simulink model "gm_sampleModel1973_sub_sub_sub"  (R2023a)
settings: Solver=VariableStepAuto  StartTime=0.0  StopTime=10.0  RelTol=1e-3
libraries: simulink x5, hdlsllib x4
settings Model: Creator=user1  LastModifiedBy=user1
settings OptimizationCC: BlockReduction=off  ConditionallyExecuteInputs=off
settings DebuggingCC: InheritedTsInSrcMsg=none

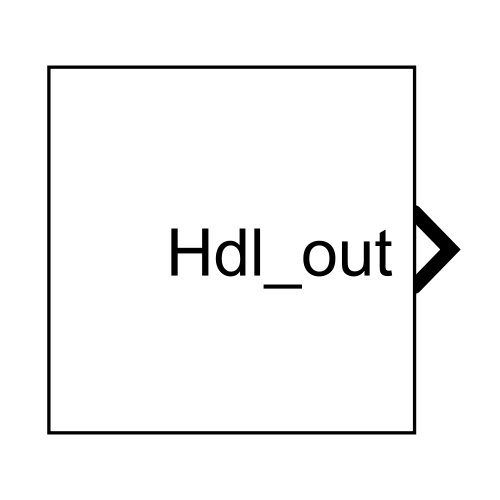
[thumbnail: Simulink's stored preview of the top-level diagram]
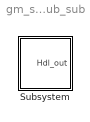
== system gm_sampleModel1973_sub_sub_sub ==
  Subsystem : Subsystem

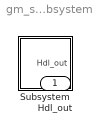
== system gm_sampleModel1973_sub_sub_sub/Subsystem ==
  Subsystem : Subsystem
  Hdl_out : Outport  OutDataTypeStr=uint8

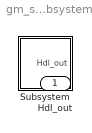
== system gm_sampleModel1973_sub_sub_sub/Subsystem/Subsystem ==
  Subsystem : Subsystem
  Hdl_out : Outport  OutDataTypeStr=uint8

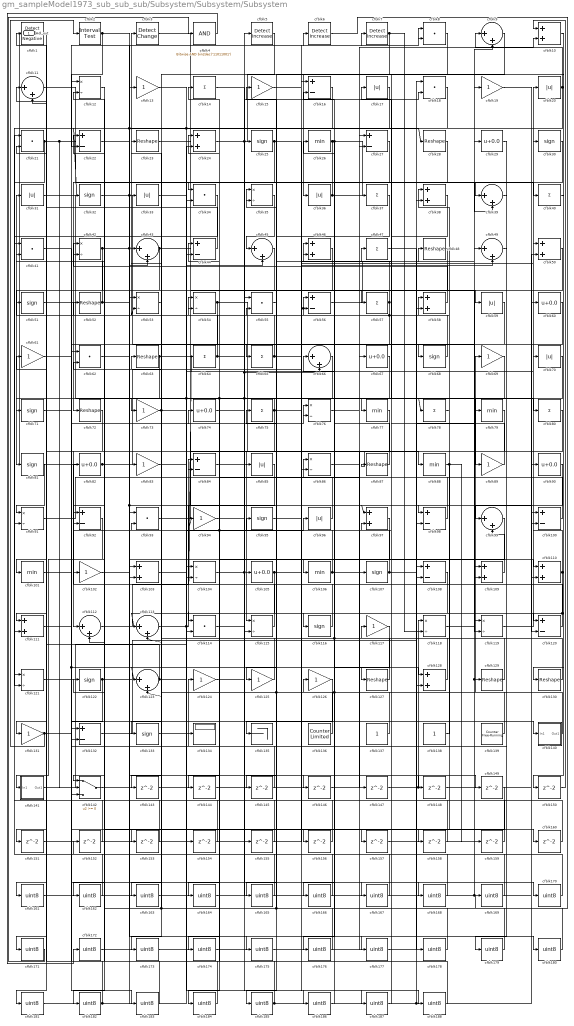
== system gm_sampleModel1973_sub_sub_sub/Subsystem/Subsystem/Subsystem ==
  cfblk1 : hdlsllib/Logic and Bit Operations/Detect Fall Negative  vinit=0  OutDataTypeStr=uint8
  cfblk{10,24,38,46,50,58,97,103,109..111,128} (12 alike) : Sum  OutDataTypeStr=uint8
  cfblk{16,22,27,44,56,84,92,98,100,108,120,132} (12 alike) : Sum  Inputs=+-  OutDataTypeStr=uint8
  cfblk{26,77,79,88,101,106} (6 alike) : MinMax  OutDataTypeStr=uint8
  cfblk{13,15,19,61,69,73,83,89,94,102,117,124..126,131} (15 alike) : Gain  OutDataTypeStr=uint8
  cfblk{12,35,42,53..54,76,86,91,104,115,118..119,121} (13 alike) : Product  Inputs=*/  OutDataTypeStr=uint8  RndMeth=Zero  SaturateOnIntegerOverflow=on
  cfblk{29,60,67,74,82,90,105} (7 alike) : Bias  Bias=0.0  SaturateOnIntegerOverflow=off
  cfblk{25,30,32,51,68,71,81,95,107,116,122,133} (12 alike) : Signum
  cfblk{9,11,39,43,45,49,66,99,112..113,123} (11 alike) : Sum  Inputs=|++  OutDataTypeStr=uint8
  cfblk{8,18,21,34,41,55,62,93,114} (9 alike) : DotProduct  OutDataTypeStr=uint8
  cfblk{23,28,48,52,63,72,87,127,129..130} (10 alike) : Reshape
  cfblk134 : Display
  cfblk135 : Terminator
  cfblk136 : hdlsllib/Sources/Counter Limited  uplimit=7  tsamp=-1
  cfblk137 : Constant  OutDataTypeStr=uint8  SampleTime=-1
  cfblk138 : Constant  OutDataTypeStr=uint8  SampleTime=-1
  cfblk139 : hdlsllib/Sources/Counter Free-Running  NumBits=16  tsamp=-1
  cfblk{14,37,40,47,57,64..65,75,78,80} (10 alike) : Sum  Inputs=+  OutDataTypeStr=uint8
  cfblk140 : Subsystem
      settings: LibrarySourceBlock=|
      | hdlsllib/Ports &
      | Subsystems/Subsystem
  cfblk141 : Subsystem
      settings: LibrarySourceBlock=|
      | hdlsllib/Ports &
      | Subsystems/Subsystem
  cfblk142 : Switch  OutDataTypeStr=uint8  SaturateOnIntegerOverflow=off  InputSameDT=off
  cfblk{143..160} (18 alike) : Delay  SampleTime=1
  cfblk{161..188} (28 alike) : DataTypeConversion  OutDataTypeStr=uint8  SaturateOnIntegerOverflow=off  RndMeth=Floor
  cfblk{17,20,31,33,36,59,70,85,96} (9 alike) : Abs  OutDataTypeStr=uint8  SaturateOnIntegerOverflow=off
  cfblk2 : hdlsllib/Logic and Bit Operations/Interval Test  IntervalClosedRight=on  uplimit=0.5  IntervalClosedLeft=on  lowlimit=-0.5  OutDataTypeStr=uint8
  cfblk3 : simulink/Logic and Bit Operations/Detect Change  vinit=0  OutDataTypeStr=uint8
      settings: LibrarySourceBlock=|
      | hdlsllib/Logic and Bit
      | Operations/Detect
      | Change
  cfblk4 : simulink/Logic and Bit Operations/Bitwise Operator  logicop=AND  UseBitMask=on  BitMask=bin2dec('11011001')  BitMaskRealWorld=Stored Integer
      settings: LibrarySourceBlock=|
      | hdlsllib/Logic and Bit
      | Operations/Bitwise
      | Operator
  cfblk5 : simulink/Logic and Bit Operations/Detect Increase  vinit=0.0  OutDataTypeStr=uint8
      settings: LibrarySourceBlock=|
      | hdlsllib/Logic and Bit
      | Operations/Detect
      | Increase
  cfblk6 : simulink/Logic and Bit Operations/Detect Increase  vinit=0.0  OutDataTypeStr=uint8
      settings: LibrarySourceBlock=|
      | hdlsllib/Logic and Bit
      | Operations/Detect
      | Increase
  cfblk7 : simulink/Logic and Bit Operations/Detect Increase  vinit=0.0  OutDataTypeStr=uint8
      settings: LibrarySourceBlock=|
      | hdlsllib/Logic and Bit
      | Operations/Detect
      | Increase
  Hdl_out : Outport  OutDataTypeStr=uint8
  wires:
  cfblk188/1 -> cfblk14/1
  cfblk187/1 -> cfblk97/2
  cfblk14/1 -> cfblk187/1
  cfblk186/1 -> cfblk126/1
  cfblk103/1 -> cfblk186/1
  cfblk185/1 -> cfblk108/2, cfblk60/1, cfblk62/1
  cfblk184/1 -> cfblk12/2
  cfblk183/1 -> cfblk12/1
  cfblk61/1 -> cfblk183/1
  cfblk182/1 -> cfblk154/1, cfblk21/2
  cfblk181/1 -> cfblk13/1
  cfblk72/1 -> cfblk181/1
  cfblk180/1 -> cfblk93/1, cfblk113/2, cfblk35/2
  cfblk179/1 -> cfblk47/1
  cfblk49/1 -> cfblk179/1
  cfblk178/1 -> cfblk152/1
  cfblk47/1 -> cfblk178/1
  cfblk177/1 -> cfblk117/1
  cfblk94/1 -> cfblk177/1
  cfblk176/1 -> cfblk63/1
  cfblk117/1 -> cfblk176/1
  cfblk175/1 -> cfblk27/2
  cfblk174/1 -> cfblk27/1
  cfblk108/1 -> cfblk174/1
  cfblk173/1 -> cfblk114/2
  cfblk27/1 -> cfblk173/1
  cfblk172/1 -> cfblk108/1
  cfblk4/1 -> cfblk172/1
  cfblk171/1 -> cfblk4/1
  cfblk45/1 -> cfblk171/1
  cfblk170/1 -> cfblk41/2
  cfblk33/1 -> cfblk170/1
  cfblk169/1 -> cfblk41/1
  cfblk6/1 -> cfblk169/1
  cfblk168/1 -> cfblk51/1
  cfblk41/1 -> cfblk168/1
  cfblk167/1 -> cfblk55/2
  cfblk166/1 -> cfblk55/1
  cfblk60/1 -> cfblk166/1
  cfblk165/1 -> cfblk122/1
  cfblk55/1 -> cfblk165/1
  cfblk164/1 -> cfblk5/1
  cfblk70/1 -> cfblk164/1
  cfblk163/1 -> cfblk19/1, cfblk129/1, cfblk90/1
  cfblk162/1 -> cfblk1/1
  cfblk149/1 -> cfblk162/1
  cfblk161/1 -> cfblk67/1
  cfblk1/1 -> cfblk161/1
  cfblk160/1 -> cfblk75/1
  cfblk159/1 -> cfblk119/1
  cfblk158/1 -> cfblk104/1
  cfblk157/1 -> cfblk9/2
  cfblk156/1 -> cfblk103/1
  cfblk97/1 -> cfblk156/1
  cfblk155/1 -> cfblk121/1
  cfblk124/1 -> cfblk155/1
  cfblk154/1 -> cfblk93/2
  cfblk153/1 -> cfblk53/1
  cfblk50/1 -> cfblk153/1
  cfblk152/1 -> cfblk21/1
  cfblk151/1 -> cfblk16/1
  cfblk150/1 -> cfblk10/1
  cfblk40/1 -> cfblk150/1
  cfblk83/1 -> cfblk149/1
  cfblk148/1 -> cfblk100/1
  cfblk147/1 -> cfblk18/1
  cfblk86/1 -> cfblk147/1
  cfblk146/1 -> cfblk58/2
  cfblk145/1 -> cfblk132/1
  cfblk37/1 -> cfblk145/1
  cfblk144/1 -> cfblk109/2
  cfblk99/1 -> cfblk144/1
  cfblk143/1 -> cfblk98/2
  cfblk48/1 -> cfblk143/1
  cfblk16/1 -> cfblk121/2
  cfblk75/1 -> cfblk71/1, cfblk101/1, cfblk188/1
  cfblk106/1 -> cfblk22/1, cfblk10/2
  cfblk100/1 -> cfblk56/1, cfblk56/2
  cfblk58/1 -> cfblk42/1
  cfblk78/1 -> cfblk58/1
  cfblk111/1 -> cfblk8/1
  cfblk22/1 -> cfblk6/1
  cfblk59/1 -> cfblk132/2
  cfblk125/1 -> cfblk94/1, cfblk44/1
  cfblk35/1 -> cfblk45/1
  cfblk142/1 -> cfblk118/1, cfblk50/2
  cfblk74/1 -> cfblk88/1
  cfblk71/1 -> cfblk140/1(In1)
  cfblk69/1 -> cfblk92/1, cfblk184/1
  cfblk91/1 -> cfblk37/1
  cfblk122/1 -> cfblk127/1, cfblk142/3
  cfblk2/1 -> cfblk28/1, cfblk167/1, cfblk22/2
  cfblk13/1 -> cfblk180/1
  cfblk15/1 -> cfblk7/1
  cfblk44/1 -> cfblk11/2
  cfblk68/1 -> cfblk16/2
  cfblk129/1 -> cfblk86/1
  cfblk121/1 -> cfblk43/2
  cfblk67/1 -> cfblk104/2, cfblk142/1
  cfblk53/1 -> cfblk23/1
  cfblk38/1 -> cfblk57/1
  cfblk34/1 -> cfblk91/2
  cfblk76/1 -> cfblk80/1
  cfblk42/1 -> cfblk8/2, cfblk146/1, cfblk111/1
  cfblk127/1 -> cfblk26/1, cfblk54/1
  cfblk18/1 -> cfblk65/1
  cfblk21/1 -> cfblk39/2, cfblk142/2, cfblk111/2
  cfblk19/1 -> cfblk120/2
  cfblk95/1 -> cfblk50/1
  cfblk107/1 -> cfblk79/1, cfblk42/2
  cfblk133/1 -> cfblk70/1
  cfblk118/1 -> cfblk49/1
  cfblk56/1 -> cfblk29/1
  cfblk132/1 -> cfblk38/2
  cfblk30/1 -> cfblk102/1
  cfblk20/1 -> cfblk9/1, cfblk151/1
  cfblk11/1 -> cfblk83/1
  cfblk131/1 -> cfblk2/1, cfblk74/1
  cfblk101/1 -> cfblk123/1, cfblk160/1
  cfblk126/1 -> cfblk185/1
  cfblk137/1 -> cfblk43/1
  cfblk17/1 -> cfblk32/1, cfblk34/2
  cfblk104/1 -> cfblk18/2, cfblk66/2, cfblk128/1
  cfblk25/1 -> cfblk73/1, cfblk128/2
  cfblk115/1 -> cfblk82/1
  cfblk120/1 -> cfblk113/1, cfblk92/2
  cfblk57/1 -> cfblk106/1, cfblk53/2, cfblk35/1
  cfblk109/1 -> cfblk99/2
  cfblk102/1 -> cfblk76/2
  cfblk12/1 -> cfblk182/1
  cfblk123/1 -> cfblk96/1, cfblk61/1
  cfblk88/1 -> cfblk158/1, cfblk159/1
  cfblk141/1(Out1) -> cfblk24/2
  cfblk82/1 -> cfblk48/1, Hdl_out/1
  cfblk73/1 -> cfblk33/1, cfblk123/2, cfblk45/2
  cfblk116/1 -> cfblk84/2
  cfblk85/1 -> cfblk114/1
  cfblk93/1 -> cfblk25/1
  cfblk32/1 -> cfblk109/1, cfblk110/1
  cfblk52/1 -> cfblk11/1, cfblk175/1
  cfblk46/1 -> cfblk112/2
  cfblk112/1 -> cfblk84/1
  cfblk23/1 -> cfblk68/1
  cfblk26/1 -> cfblk116/1, cfblk110/2, cfblk44/2
  cfblk138/1 -> cfblk38/1
  cfblk54/1 -> cfblk107/1, cfblk133/1
  cfblk140/1(Out1) -> cfblk46/2, cfblk54/2
  cfblk96/1 -> cfblk24/1
  cfblk5/1 -> cfblk163/1
  cfblk9/1 -> cfblk77/1
  cfblk113/1 -> cfblk64/1, cfblk148/1
  cfblk87/1 -> cfblk66/1
  cfblk105/1 -> cfblk115/2, cfblk49/2
  cfblk80/1 -> cfblk112/1
  cfblk130/1 -> cfblk52/1
  cfblk92/1 -> cfblk141/1(In1)
  cfblk8/1 -> cfblk36/1
  cfblk51/1 -> cfblk134/1
  cfblk43/1 -> cfblk81/1, cfblk119/2
  cfblk110/1 -> cfblk30/1, cfblk135/1
  cfblk128/1 -> cfblk15/1
  cfblk98/1 -> cfblk46/1
  cfblk114/1 -> cfblk76/1
  cfblk79/1 -> cfblk105/1
  cfblk77/1 -> cfblk87/1
  cfblk62/1 -> cfblk97/1, cfblk157/1
  cfblk66/1 -> cfblk131/1
  cfblk136/1 -> cfblk95/1, cfblk62/2
  cfblk81/1 -> cfblk91/1
  cfblk29/1 -> cfblk59/1
  cfblk7/1 -> cfblk125/1, cfblk118/2
  cfblk65/1 -> cfblk3/1, cfblk100/2
  cfblk10/1 -> cfblk120/1
  cfblk64/1 -> cfblk78/1, cfblk86/2, cfblk31/1
  cfblk24/1 -> cfblk130/1, cfblk40/1
  cfblk119/1 -> cfblk20/1
  cfblk89/1 -> cfblk17/1
  cfblk39/1 -> cfblk99/1
  cfblk31/1 -> cfblk89/1
  cfblk63/1 -> cfblk85/1, cfblk103/2
  cfblk84/1 -> cfblk115/1
  cfblk90/1 -> cfblk124/1
  cfblk139/1 -> cfblk69/1
  cfblk28/1 -> cfblk72/1
  cfblk36/1 -> cfblk39/1, cfblk34/1
  cfblk3/1 -> cfblk98/1

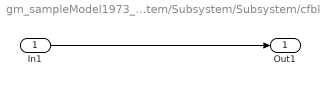
== system gm_sampleModel1973_sub_sub_sub/Subsystem/Subsystem/Subsystem/cfblk140 ==
  In1 : Inport
  Out1 : Outport
  wires:
  In1/1 -> Out1/1

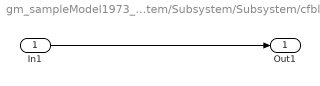
== system gm_sampleModel1973_sub_sub_sub/Subsystem/Subsystem/Subsystem/cfblk141 ==
  In1 : Inport
  Out1 : Outport
  wires:
  In1/1 -> Out1/1
